simulink model "VoltageSourceSimulation"  (R2015b)
settings: Solver=ode45  StartTime=0.0  StopTime=1  RelTol=1e-3
values from neighbouring files (symbols this model uses):
  c2_val = 200e-6    (= 0.0002)    [VoltageSourceController.m]    (also in main.m = 1e-06)
  fs2 = 2e3    (= 2000)    [VoltageSourceController.m]
  l2_val = 50e-4    (= 0.005)    [VoltageSourceController.m]    (also in main.m = 1e-08)
  r_val = 1    [CurrentSourceController.m]    (also in VoltageSourceController.m; main.m)
  Vd_val = 100    [CurrentSourceController.m]    (also in VoltageSourceController.m = 8; main.m = 110)
libraries: powerlib x11, simulink x1, simulink_extras x1
settings Model: SimulationMode=accelerator  Creator=Akshay  LastModifiedBy=Akshay
settings SolverCC: ZeroCrossAlgorithm=Adaptive

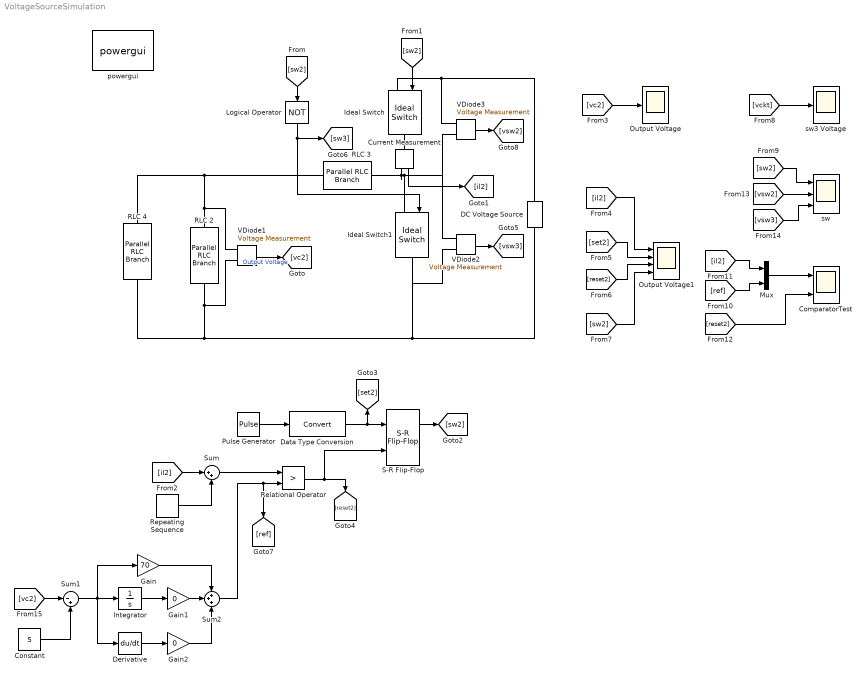
== system VoltageSourceSimulation ==
  " RLC 2" : powerlib/Elements/Parallel RLC Branch  LConnTagsString=a  RConnTagsString=__new0  BranchType=C  Resistance=1  Inductance=1e-3  SetiL0=off  InitialCurrent=0  Capacitance=c2_val  Setx0=off  InitialVoltage=50  Measurements=None
  " RLC 3" : powerlib/Elements/Parallel RLC Branch  LConnTagsString=a  RConnTagsString=__new0  BranchType=L  Resistance=50  Inductance=l2_val  SetiL0=on  InitialCurrent=0  Capacitance=0.3e-6  Setx0=off  InitialVoltage=0  Measurements=None
  " RLC 4" : powerlib/Elements/Parallel RLC Branch  LConnTagsString=a  RConnTagsString=__new0  BranchType=R  Resistance=r_val  Inductance=1e-3  SetiL0=off  InitialCurrent=0  Capacitance=0.1e-6  Setx0=off  InitialVoltage=0  Measurements=None
  ComparatorTest : Scope  NumInputPorts=2
  Constant : Constant  Value=5
  Current Measurement : powerlib/Measurements/Current Measurement  PhasorSimulation=off  OutputType=Complex  PSBequivalent=0
  DC Voltage Source : powerlib/Electrical Sources/DC Voltage Source  Amplitude=Vd_val  Measurements=Voltage
  Data Type Conversion : DataTypeConversion
  Derivative : Derivative
  Gain : Gain  Gain=70
  Gain1 : Gain  Gain=0
  Gain2 : Gain  Gain=0
  Ideal Switch : powerlib/Power Electronics/Ideal Switch  Ron=1e-7  Lon=0  IC=0  Rs=inf  Cs=inf  Measurements=off
  Ideal Switch1 : powerlib/Power Electronics/Ideal Switch  Ron=1e-7  Lon=0  IC=1  Rs=inf  Cs=inf  Measurements=off
  Integrator : Integrator
  Logical Operator : Logic  Operator=NOT  AllPortsSameDT=off  OutDataTypeStr=boolean
  Mux : Mux  Inputs=2
  Output Voltage : Scope
  Output Voltage1 : Scope  NumInputPorts=4
  Pulse Generator : DiscretePulseGenerator  PulseType=Time based  Period=1/fs2  PulseWidth=5
  Relational Operator : RelationalOperator  Operator=>  OutDataTypeStr=boolean
  Repeating Sequence : simulink/Sources/Repeating Sequence  rep_seq_t=[0 1/fs2]  rep_seq_y=[0 0]
  S-R Flip-Flop : simulink_extras/Flip Flops/S-R Flip-Flop  initial_condition=0
  Sum : Sum  Inputs=|++
  Sum1 : Sum  Inputs=|-+
  Sum2 : Sum  Inputs=+++
  VDiode1 : powerlib/Measurements/Voltage Measurement  PhasorSimulation=off  OutputType=Complex  PSBequivalent=0
  VDiode2 : powerlib/Measurements/Voltage Measurement  PhasorSimulation=off  OutputType=Complex  PSBequivalent=0
  VDiode3 : powerlib/Measurements/Voltage Measurement  PhasorSimulation=off  OutputType=Complex  PSBequivalent=0
  powergui : powerlib/powergui  Priority=1  SimulationMode=Continuous  SolverType=Backward Euler  SampleTime=5e-07  frequency=60  SPID=on  DisableSnubberDevices=off  DisableRonSwitches=off  DisableVfSwitches=off  SwTol=0  DisplayEquations=off  Interpol=off  ExternalGateDelay=off  methode=off  Ts=0  FunctionMessages=off  echomessages=off  HookPort=off  EnableUseOfTLC=off  x0status=zero  frequencyindice=0  Pbase=100e6  ErrMax=1e-4  Iterations=50  UnitsV=kV  UnitsW=MW  buscounter=0  RestoreLinks=warning  ResistiveCurrentMeasurement=off  Frange=[0:2:500]  Ylog=off  Xlog=on  ShowGrid=off  save=off  variable=ZData  structure=ScopeData  ZoomFFT=off  StartTime=0.0  cycles=5  DisplayStyle=2  fundamental=50  FreqAxis=off  MaxFrequency=50000  frequencyindicesteady=1  RmsSteady=1  display=off
  sw : Scope  NumInputPorts=3
  sw3 Voltage : Scope
  wires:
  VDiode1/1 -> [vc2]  "Output Voltage"
  Current Measurement/1 -> [il2]
  Pulse Generator/1 -> Data Type Conversion/1
  Data Type Conversion/1 -> S-R Flip-Flop/1, [set2]
  [sw2] -> Logical Operator/1
  Relational Operator/1 -> S-R Flip-Flop/2, [reset2]
  [vc2] -> Output Voltage/1
  [il2] -> Output Voltage1/1
  [set2] -> Output Voltage1/2
  [reset2] -> Output Voltage1/3
  [sw2] -> Output Voltage1/4
  VDiode2/1 -> [vsw3]
  [vckt] -> sw3 Voltage/1
  [sw2] -> sw/1
  S-R Flip-Flop/1 -> [sw2]
  Logical Operator/1 -> [sw3], Ideal Switch1/1
  [sw2] -> Ideal Switch/1
  [il2] -> Mux/1
  [ref] -> Mux/2
  Mux/1 -> ComparatorTest/1
  [reset2] -> ComparatorTest/2
  VDiode3/1 -> [vsw2]
  [vsw3] -> sw/3
  [vsw2] -> sw/2
  [il2] -> Sum/1
  Repeating Sequence/1 -> Sum/2
  Sum/1 -> Relational Operator/1
  [vc2] -> Sum1/1
  Constant/1 -> Sum1/2
  Sum1/1 -> Derivative/1, Gain/1, Integrator/1
  Integrator/1 -> Gain1/1
  Gain1/1 -> Sum2/2
  Gain/1 -> Sum2/1
  Sum2/1 -> Relational Operator/2, [ref]
  Derivative/1 -> Gain2/1
  Gain2/1 -> Sum2/3
  connections:
  " RLC 3"/RConn1 -- Current Measurement/RConn1 -- VDiode3/LConn2 -- VDiode2/LConn1 -- Ideal Switch1/LConn1
  " RLC 2"/RConn1 -- VDiode1/LConn2 -- Ideal Switch1/RConn1 -- VDiode2/LConn2 -- DC Voltage Source/LConn1 -- " RLC 4"/RConn1
  " RLC 2"/LConn1 -- VDiode1/LConn1 -- " RLC 4"/LConn1 -- " RLC 3"/LConn1
  Ideal Switch/LConn1 -- VDiode3/LConn1 -- DC Voltage Source/RConn1
  Current Measurement/LConn1 -- Ideal Switch/RConn1
